simulink model "MyMOAB"  (R2021a)
settings: Solver=ode23t  StartTime=0.0  StopTime=Inf  RelTol=1e-3  AbsTol=1e-3
values from neighbouring files (symbols this model uses):
  ball_mass = DEFAULT_BALL_MASS    (= 0.0027)    [MOAB_PARAMS.m]
  ball_moi = calcMOI(ball_radius,ball_shell,ball_mass)    [MOAB_PARAMS.m]
  ball_radius = DEFAULT_BALL_RADIUS    (= 0.02)    [MOAB_PARAMS.m]
  ball_shell = DEFAULT_BALL_SHELL    (= 0.0002)    [MOAB_PARAMS.m]
  DEFAULT_BALL_NOISE = 0.0005    [MOAB_PARAMS.m]
  DEFAULT_GRAVITY = 9.81    [MOAB_PARAMS.m]
  DEFAULT_PLATE_NOISE = 0.0    (= 0)    [MOAB_PARAMS.m]
  DEFAULT_SIMULATION_RATE = 0.2    [MOAB_PARAMS.m]
  DEFAULT_VEL_NOISE = 0.0001    [MOAB_PARAMS.m]
  MAX_ITER = Inf    (= inf)    [MOAB_PARAMS.m]
  noise_mean = 0    [MOAB_PARAMS.m]
  noise_variance = 0.333    [MOAB_PARAMS.m]
  obstacle_radius = DEFAULT_OBSTACLE_RADIUS    (= 0)    [MOAB_PARAMS.m]
  plate_pos_z0 = DEFAULT_PLATE_HEIGHT    (= 0.02)    [MOAB_PARAMS.m]
  plate_radius = DEFAULT_PLATE_RADIUS    (= 0.1125)    [MOAB_PARAMS.m]
  s = 0.1732    [MOAB_PARAMS.m]
  target_pos_x = 0    [MOAB_PARAMS.m]
  target_pos_y = 0    [MOAB_PARAMS.m]
  tilt_acc = DEFAULT_PLATE_ANGULAR_ACCEL    [MOAB_PARAMS.m]
  tilt_limit = DEFAULT_PLATE_ANGLE_LIMIT    [MOAB_PARAMS.m]
  tilt_max_vel = DEFAULT_PLATE_MAX_ANGULAR_VELOCITY    [MOAB_PARAMS.m]
  tilt_x0 = deg2rad(0)    [MOAB_PARAMS.m]
  tilt_y0 = deg2rad(0)    [MOAB_PARAMS.m]
  TIME_DELTA = DEFAULT_SIMULATION_RATE    (= 0.2)    [MOAB_PARAMS.m]
  z_offset = 0.0328538    [MOAB_PARAMS.m]
undefined symbols (not defined in the file or in its folder): smiData, X, Y, Z
libraries: sm_lib x119, nesl_utility x21, simulink x1
(part 1 of 4)
settings Model: Creator=abiswas  LastModifiedBy=dbnun
settings SolverCC: AlgebraicLoopSolver=TrustRegion
settings DebuggingCC: InheritedTsInSrcMsg=none  SFMachineParentedDataDiag=warning
settings SimscapeCC: SimscapeLogType=all
settings DiagnosticsConfigSet: SimMechanicsUnsatisfiedHighPriorityTargets=none
settings ExplorerConfigSet: InternalSimMechanicsExplorerSettings="<ExplorerConfiguration><canonicalview>default</canonicalview><AnimationSetting><BasePlaybackSpeed>1.0</BasePlaybackSpeed><PlaybackSpeedFactor>1.0</PlaybackSpeedFactor></AnimationSetting><TilePanel><TileInfo><Tiles Columns=\"1\" Count=\"2\" Rows=\"2\"><Column Weight=\"1\"/><Row Weight=\"0.5678\"/><Row Weight=\"0.4322\"/><Tile Height=\"1\" Width=\"1\" X=\"0\" Y=\"0\"/><Tile Height=\"1\" Width=\"1\" X=\"0\" Y=\"1\"/></Tiles></TileInfo><SceneInfo><SceneViewer><BGColor><R>1</R><G>1</G><B>1</B></BGColor><Camera><DoPerspective>off</DoPerspective><Position><X>-0.0080012764069667501</X><Y>-0.00465270619968879105</Y><Z>1.03071236736211413</Z></Position><Center><X>-0.0080012764069667501</X><Y>-0.00465270619968879105</Y><Z>0.0307123673621141347</Z></Center><Up><X>-0.84666783086952091</X><Y>-0.532121775696785759</Y><Z>0</Z></Up><ViewLimDist>1</ViewLimDist><YLim>0.139428062443435197</YLim><XLim>0.213694846724530263</XLim></Camera></SceneViewer><SceneViewer><BGColor><R>1</R><G>1</G><B>1</B></BGColor><Camera><DoPerspective>off</DoPerspective><Position><X>0.994386182454623402</X><Y>0.0608673913546442444</Y><Z>0.0679676248852747467</Z></Position><Center><X>-0.00298892093291726986</X><Y>0.00143103908732779002</Y><Z>0.0266127802857842946</Z></Center><Up><X>-0.040438631297503691</X><Y>-0.0165365771902967751</Y><Z>0.999045173509994111</Z></Up><ViewLimDist>1</ViewLimDist><YLim>0.077297016049004505</YLim><XLim>0.156048545840866637</XLim></Camera></SceneViewer></SceneInfo></TilePanel><MechEditorPanel><Cameras/><GfxPanelCameraMap/><VideoCreator><PlaybackSpeedRatio>1.0</PlaybackSpeedRatio><FrameRate>30</FrameRate><VideoFormat>Motion JPEG AVI</VideoFormat><FrameSize>auto</FrameSize></VideoCreator></MechEditorPanel></ExplorerConfiguration>"

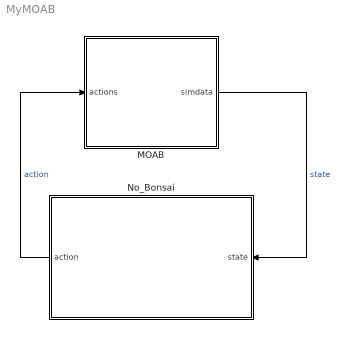
== system MyMOAB ==
  MOAB : Subsystem
      mask Display: image('MOAB_Full_IMAGE.png')
  No_Bonsai : Subsystem  VariantControl=Sinusoid
  wires:
  MOAB/1(simdata) -> No_Bonsai/1(state)  "state"
  No_Bonsai/1(action) -> MOAB/1(actions)  "action"

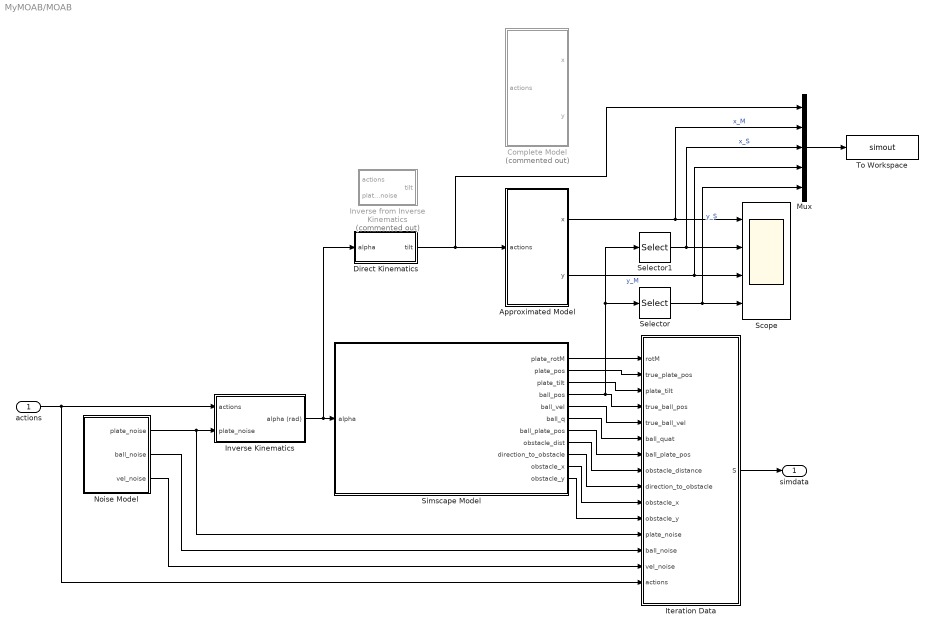
== system MyMOAB/MOAB ==
  actions : Inport
  Approximated Model : Subsystem
  Complete Model : Subsystem  Commented=on
  Direct Kinematics : Subsystem
  Inverse Kinematics : Subsystem
  Inverse from Inverse Kinematics : Subsystem  Commented=on
  Iteration Data : Subsystem  VariantControl=Choice
  Mux : Mux  Inputs=5
  Noise Model : Subsystem  Variant=on  VariantControlMode=label  LabelModeActiveChoice=Zero  mask{VChoice=Zero noise}
      mask prompts: VChoice "Noise model"
      mask init:
      | simulationStatus =  get_param(bdroot,'SimulationStatus');
      | 
      | % The active variant can only be modified at edit-time or very early during
      | % the simulink compile stage. 
      | 
      |     choice = get_param(gcb,'VChoice');
      |     vssBlk = gcb;
      |     oldVariant = get_param(gcb,'OverrideUsingVariant');
      | 
      |     if strcmp(choice,'Zero noise')
      | 
      |         set_param(vssBlk, 'OverrideUsingVariant', 'Zero');
      |     else
      | 
      |         set_param(vssBlk, 'OverrideUsingVariant', 'Gaussian');
      |     end
      mask TypeOptions VChoice: Zero noise | Gaussian noise
      mask DialogControl DescTextVar Prompt: Select a noise model for ball and plate states.
  Scope : Scope  NumInputPorts=4
  Selector : Selector  InputPortWidth=3  IndexOptions=Index vector (dialog)  Indices=[2]  OutputSizes=1
  Selector1 : Selector  InputPortWidth=3  IndexOptions=Index vector (dialog)  Indices=[1]  OutputSizes=1
  Simscape Model : Subsystem
      mask Display: image('MOAB_Full_IMAGE_small.png')
  To Workspace : ToWorkspace  VariableName=simout  SaveFormat=Timeseries  SampleTime=-1
  simdata : Outport
  wires:
  Inverse Kinematics/1(alpha (rad)) -> Direct Kinematics/1(alpha), Simscape Model/1(alpha)
  Noise Model/1(plate_noise) -> Inverse Kinematics/2(plate_noise), Iteration Data/12(plate_noise)
  Iteration Data/1(S) -> simdata/1
  Noise Model/2(ball_noise) -> Iteration Data/13(ball_noise)
  Noise Model/3(vel_noise) -> Iteration Data/14(vel_noise)
  Simscape Model/7(ball_plate_pos) -> Iteration Data/7(ball_plate_pos)
  Simscape Model/6(ball_q) -> Iteration Data/6(ball_quat)
  Simscape Model/5(ball_vel) -> Iteration Data/5(true_ball_vel)
  Simscape Model/4(ball_pos) -> Selector1/1, Selector/1, Iteration Data/4(true_ball_pos)
  Simscape Model/2(plate_pos) -> Iteration Data/2(true_plate_pos)
  Simscape Model/1(plate_rotM) -> Iteration Data/1(rotM)
  Simscape Model/8(obstacle_dist) -> Iteration Data/8(obstacle_distance)
  Simscape Model/3(plate_tilt) -> Iteration Data/3(plate_tilt)
  Simscape Model/9(direction_to_obstacle) -> Iteration Data/9(direction_to_obstacle)
  Simscape Model/10(obstacle_x) -> Iteration Data/10(obstacle_x)
  Simscape Model/11(obstacle_y) -> Iteration Data/11(obstacle_y)
  Selector/1 -> Mux/5, Scope/4  "y_S"
  Selector1/1 -> Mux/3, Scope/2  "x_S"
  actions/1 -> Iteration Data/15(actions), Inverse Kinematics/1(actions)
  Approximated Model/2(y) -> Mux/4, Scope/3  "y_M"
  Approximated Model/1(x) -> Mux/2, Scope/1  "x_M"
  Direct Kinematics/1(tilt) -> Mux/1, Approximated Model/1(actions)
  Mux/1 -> To Workspace/1

== system MyMOAB/No_Bonsai ==
  state : Inport
  Constant1 : Constant  Value=false
  "Sinusoidal " : Subsystem
  Stop Simulation1 : Stop
  action : Outport
  wires:
  Constant1/1 -> "Sinusoidal "/2(halted)
  "Sinusoidal "/2(reset) -> Stop Simulation1/1
  state/1 -> "Sinusoidal "/1(state)
  "Sinusoidal "/1(actions) -> action/1

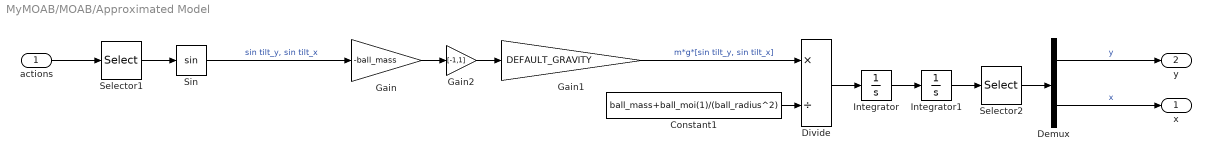
== system MyMOAB/MOAB/Approximated Model ==
  actions : Inport
  Constant1 : Constant  Value=ball_mass+ball_moi(1)/(ball_radius^2)
  Demux : Demux  Outputs=2
  Divide : Product  Inputs=*/
  Gain : Gain  Gain=-ball_mass
  Gain1 : Gain  Gain=DEFAULT_GRAVITY
  Gain2 : Gain  Gain=[-1,1]
  Integrator : Integrator
  Integrator1 : Integrator
  Selector1 : Selector  InputPortWidth=2  IndexOptions=Index vector (dialog)  Indices=[2 1]  OutputSizes=1
  Selector2 : Selector  InputPortWidth=2  IndexOptions=Index vector (dialog)  Indices=[2 1]  OutputSizes=1
  Sin : Trigonometry
  x : Outport
  y : Outport  Port=2
  wires:
  Divide/1 -> Integrator/1
  Integrator/1 -> Integrator1/1
  Demux/2 -> x/1  "x"
  Gain1/1 -> Divide/1  "m*g*[sin tilt_y, sin tilt_x]"
  Selector1/1 -> Sin/1
  Demux/1 -> y/1  "y"
  Integrator1/1 -> Selector2/1
  Selector2/1 -> Demux/1
  actions/1 -> Selector1/1
  Constant1/1 -> Divide/2
  Sin/1 -> Gain/1  "sin tilt_y, sin tilt_x"
  Gain/1 -> Gain2/1
  Gain2/1 -> Gain1/1

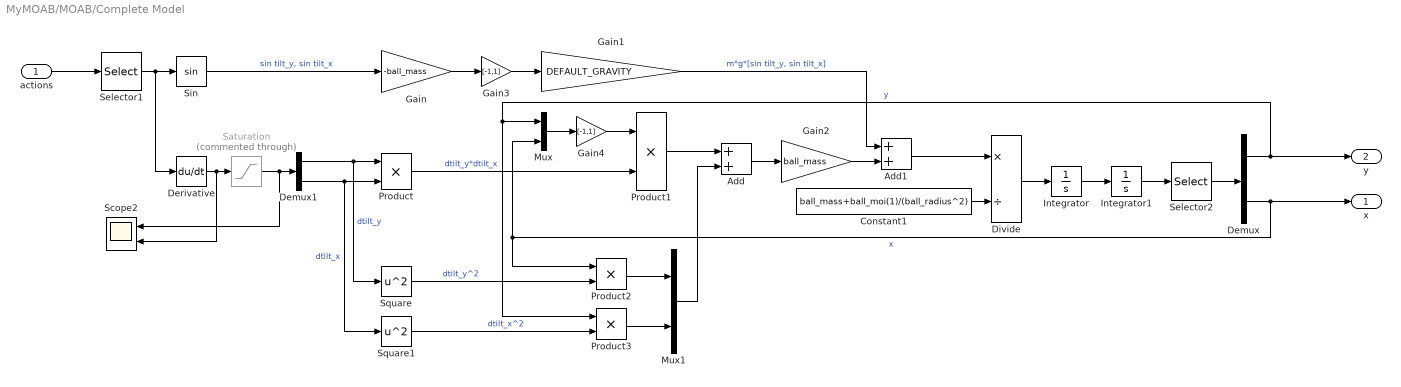
== system MyMOAB/MOAB/Complete Model ==
  actions : Inport
  Add : Sum
  Add1 : Sum
  Constant1 : Constant  Value=ball_mass+ball_moi(1)/(ball_radius^2)
  Demux : Demux  Outputs=2
  Demux1 : Demux  Outputs=2
  Derivative : Derivative
  Divide : Product  Inputs=*/
  Gain : Gain  Gain=-ball_mass
  Gain1 : Gain  Gain=DEFAULT_GRAVITY
  Gain2 : Gain  Gain=ball_mass
  Gain3 : Gain  Gain=[-1,1]
  Gain4 : Gain  Gain=[-1,1]
  Integrator : Integrator
  Integrator1 : Integrator
  Mux : Mux  Inputs=2
  Mux1 : Mux  Inputs=2
  Product{,1..3} (4 alike) : Product
  Saturation : Saturate  Commented=through  UpperLimit=50  LowerLimit=-50
  Scope2 : Scope  NumInputPorts=2
  Selector1 : Selector  InputPortWidth=2  IndexOptions=Index vector (dialog)  Indices=[2 1]  OutputSizes=1
  Selector2 : Selector  InputPortWidth=2  IndexOptions=Index vector (dialog)  Indices=[2 1]  OutputSizes=1
  Sin : Trigonometry
  Square : Math  Operator=square  SaturateOnIntegerOverflow=on
  Square1 : Math  Operator=square  SaturateOnIntegerOverflow=on
  x : Outport
  y : Outport  Port=2
  wires:
  Demux1/2 -> Square1/1, Product/2  "dtilt_x"
  Add/1 -> Gain2/1
  Square/1 -> Product2/2  "dtilt_y^2"
  Square1/1 -> Product3/2  "dtilt_x^2"
  Mux1/1 -> Add/2
  Derivative/1 -> Scope2/2, Saturation/1
  Product2/1 -> Mux1/1
  Gain2/1 -> Add1/2
  Divide/1 -> Integrator/1
  Integrator/1 -> Integrator1/1
  Product1/1 -> Add/1
  Demux1/1 -> Square/1, Product/1  "dtilt_y"
  Add1/1 -> Divide/1
  Demux/2 -> x/1, Mux/2, Product2/1  "x"
  Gain1/1 -> Add1/1  "m*g*[sin tilt_y, sin tilt_x]"
  Gain/1 -> Gain3/1
  Mux/1 -> Gain4/1
  Product/1 -> Product1/2  "dtilt_y*dtilt_x"
  Saturation/1 -> Scope2/1, Demux1/1
  Selector1/1 -> Sin/1, Derivative/1
  Demux/1 -> y/1, Product3/1, Mux/1  "y"
  Integrator1/1 -> Selector2/1
  Selector2/1 -> Demux/1
  actions/1 -> Selector1/1
  Constant1/1 -> Divide/2
  Product3/1 -> Mux1/2
  Sin/1 -> Gain/1  "sin tilt_y, sin tilt_x"
  Gain3/1 -> Gain1/1
  Gain4/1 -> Product1/1

== system MyMOAB/MOAB/Direct Kinematics ==
  alpha : Inport
  Constant : Constant  Value=plate_pos_z0+z_offset
  MATLAB Function : MATLAB Function  TreatAsAtomicUnit=on
  tilt : Outport
  wires:
  Constant/1 -> MATLAB Function/2(h)
  alpha/1 -> MATLAB Function/1(alpha)
  MATLAB Function/1(tilt) -> tilt/1

== system MyMOAB/MOAB/Inverse Kinematics ==
  note: Generate approximate servo angles from plate height and tilt angles.
  actions : Inport
  plate_noise : Inport  Port=2
  Constant : Constant  Value=plate_pos_z0+z_offset
  Convert To Tilt Angles : Gain  Gain=tilt_limit
  Demux : Demux  Outputs=2
  MATLAB Function : MATLAB Function  TreatAsAtomicUnit=on
  Reshape : Reshape
  alpha (rad) : Outport
  wires:
  Demux/2 -> MATLAB Function/3(tilt_y)  "(rad)"
  Demux/1 -> MATLAB Function/2(tilt_x)  "(rad)"
  MATLAB Function/1(alpha) -> Reshape/1
  Constant/1 -> MATLAB Function/1(plate_height)
  Reshape/1 -> alpha (rad)/1
  plate_noise/1 -> MATLAB Function/4(plate_noise)
  actions/1 -> Convert To Tilt Angles/1
  Convert To Tilt Angles/1 -> Demux/1

== system MyMOAB/MOAB/Inverse from Inverse Kinematics ==
  actions : Inport
  plate_noise : Inport  Port=2
  Convert To Tilt Angles : Gain  Gain=tilt_limit
  Sum : Sum  Inputs=|++
  tilt : Outport
  wires:
  Convert To Tilt Angles/1 -> Sum/1
  actions/1 -> Convert To Tilt Angles/1
  plate_noise/1 -> Sum/2
  Sum/1 -> tilt/1

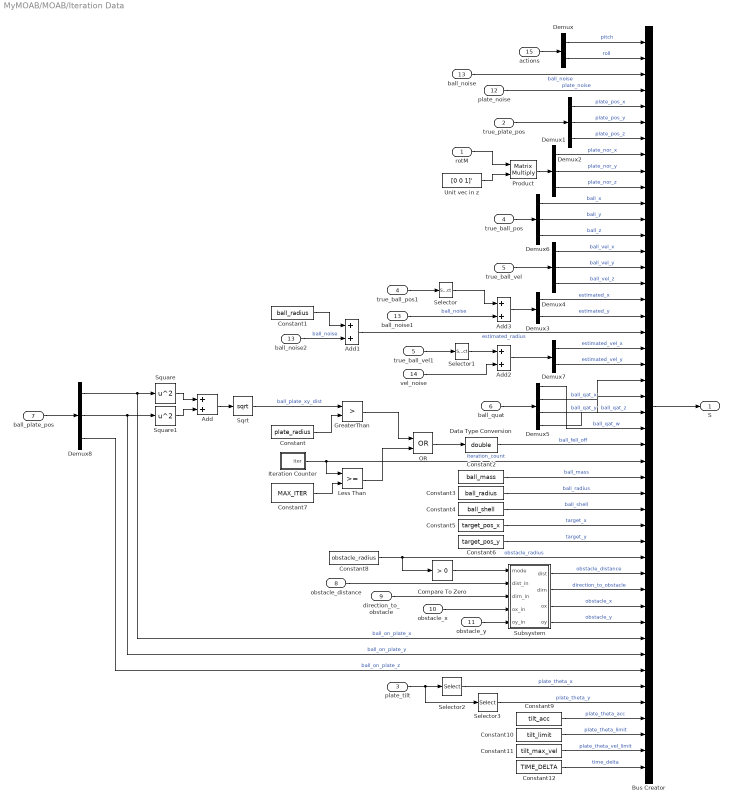
== system MyMOAB/MOAB/Iteration Data ==
  rotM : Inport
  true_plate_pos : Inport  Port=2
  plate_tilt : Inport  Port=3
  true_ball_pos : Inport  Port=4
  true_ball_vel : Inport  Port=5
  ball_quat : Inport  Port=6
  ball_plate_pos : Inport  Port=7
  obstacle_distance : Inport  Port=8
  direction_to_obstacle : Inport  Port=9
  obstacle_x : Inport  Port=10
  obstacle_y : Inport  Port=11
  plate_noise : Inport  Port=12
  ball_noise : Inport  Port=13
  vel_noise : Inport  Port=14
  actions : Inport  Port=15
  Add{,1..3} (4 alike) : Sum
  Bus Creator : BusCreator  Inputs=46
  Compare To Zero : simulink/Logic and Bit Operations/Compare To Zero  relop=>  OutDataTypeStr=boolean
  Constant : Constant  Value=plate_radius
  Constant1 : Constant  Value=ball_radius
  Constant10 : Constant  Value=tilt_limit
  Constant11 : Constant  Value=tilt_max_vel
  Constant12 : Constant  Value=TIME_DELTA
  Constant2 : Constant  Value=ball_mass
  Constant3 : Constant  Value=ball_radius
  Constant4 : Constant  Value=ball_shell
  Constant5 : Constant  Value=target_pos_x
  Constant6 : Constant  Value=target_pos_y
  Constant7 : Constant  Value=MAX_ITER
  Constant8 : Constant  Value=obstacle_radius
  Constant9 : Constant  Value=tilt_acc
  Data Type Conversion : DataTypeConversion  OutDataTypeStr=double
  Demux : Demux  Outputs=2
  Demux{1..2,4,6,8} (5 alike) : Demux  Outputs=3
  Demux3 : Demux  Outputs=2
  Demux5 : Demux
  Demux7 : Demux  Outputs=2
  GreaterThan : RelationalOperator  Operator=>  OutDataTypeStr=boolean  RndMeth=Simplest
  Iteration Counter : Subsystem
  Less Than : RelationalOperator  OutDataTypeStr=boolean  RndMeth=Simplest
  OR : Logic  Operator=OR  AllPortsSameDT=off  OutDataTypeStr=boolean
  Product : Product  Multiplication=Matrix(*)
  Selector : Selector  InputPortWidth=3  IndexOptions=Index vector (dialog)  Indices=1:2  OutputSizes=1
  Selector1 : Selector  InputPortWidth=3  IndexOptions=Index vector (dialog)  Indices=1:2  OutputSizes=1
  Selector2 : Selector  InputPortWidth=3  IndexOptions=Index vector (dialog)  Indices=1  OutputSizes=1
  Selector3 : Selector  InputPortWidth=3  IndexOptions=Index vector (dialog)  Indices=2  OutputSizes=1
  Sqrt : Sqrt  SaturateOnIntegerOverflow=on
  Square : Math  Operator=square  SaturateOnIntegerOverflow=on
  Square1 : Math  Operator=square  SaturateOnIntegerOverflow=on
  Subsystem : Subsystem
  Unit vec in z : Constant  Value=[0 0 1]'
  ball_noise1 : InportShadow  Port=13
  ball_noise2 : InportShadow  Port=13
  true_ball_pos1 : InportShadow  Port=4
  true_ball_vel1 : InportShadow  Port=5
  S : Outport
  wires:
  Demux3/2 -> Bus Creator/18  "estimated_y"
  true_ball_pos/1 -> Demux6/1
  Demux2/1 -> Bus Creator/5  "plate_pos_x"
  Demux5/3 -> Bus Creator/23  "ball_qat_y"
  Demux5/1 -> Bus Creator/25  "ball_qat_w"
  Product/1 -> Demux1/1
  Demux4/1 -> Bus Creator/14  "ball_vel_x"
  Demux5/2 -> Bus Creator/22  "ball_qat_x"
  Demux1/2 -> Bus Creator/9  "plate_nor_y"
  Demux2/3 -> Bus Creator/7  "plate_pos_z"
  Unit vec in z/1 -> Product/2
  rotM/1 -> Product/1
  Demux2/2 -> Bus Creator/6  "plate_pos_y"
  Demux/1 -> Bus Creator/1  "pitch"
  Constant10/1 -> Bus Creator/44  "plate_theta_limit"
  Add3/1 -> Demux3/1
  Iteration Counter/1(iter) -> Less Than/1, Bus Creator/27  "iteration_count"
  Subsystem/4(oy) -> Bus Creator/37  "obstacle_y"
  Demux8/3 -> Bus Creator/40  "ball_on_plate_z"
  true_ball_vel1/1 -> Selector1/1
  Demux5/4 -> Bus Creator/24  "ball_qat_z"
  Square1/1 -> Add/2
  ball_noise2/1 -> Add1/2  "ball_noise"
  Constant6/1 -> Bus Creator/32  "target_y"
  true_ball_pos1/1 -> Selector/1
  Constant5/1 -> Bus Creator/31  "target_x"
  Constant2/1 -> Bus Creator/28  "ball_mass"
  plate_noise/1 -> Bus Creator/4  "plate_noise"
  Constant/1 -> GreaterThan/2
  GreaterThan/1 -> OR/1
  Data Type Conversion/1 -> Bus Creator/26  "ball_fell_off"
  Add2/1 -> Demux7/1
  true_ball_vel/1 -> Demux4/1
  true_plate_pos/1 -> Demux2/1
  OR/1 -> Data Type Conversion/1
  Demux3/1 -> Bus Creator/17  "estimated_x"
  Demux4/2 -> Bus Creator/15  "ball_vel_y"
  Bus Creator/1 -> S/1
  Demux4/3 -> Bus Creator/16  "ball_vel_z"
  Subsystem/3(ox) -> Bus Creator/36  "obstacle_x"
  Demux6/2 -> Bus Creator/12  "ball_y"
  Less Than/1 -> OR/2
  Add/1 -> Sqrt/1
  Subsystem/2(dirn) -> Bus Creator/35  "direction_to_obstacle"
  Constant11/1 -> Bus Creator/45  "plate_theta_vel_limit"
  Demux1/3 -> Bus Creator/10  "plate_nor_z"
  Subsystem/1(dist) -> Bus Creator/34  "obstacle_distance"
  Constant3/1 -> Bus Creator/29  "ball_radius"
  Constant12/1 -> Bus Creator/46  "time_delta"
  vel_noise/1 -> Add2/2
  Selector2/1 -> Bus Creator/41  "plate_theta_x"
  Sqrt/1 -> GreaterThan/1  "ball_plate_xy_dist"
  Demux7/1 -> Bus Creator/20  "estimated_vel_x"
  Constant8/1 -> Bus Creator/33, Compare To Zero/1  "obstacle_radius"
  Square/1 -> Add/1
  actions/1 -> Demux/1
  Selector3/1 -> Bus Creator/42  "plate_theta_y"
  Demux/2 -> Bus Creator/2  "roll"
  ball_noise/1 -> Bus Creator/3  "ball_noise"
  Demux6/1 -> Bus Creator/11  "ball_x"
  plate_tilt/1 -> Selector3/1, Selector2/1
  Constant7/1 -> Less Than/2
  Selector/1 -> Add3/1
  Constant9/1 -> Bus Creator/43  "plate_theta_acc"
  Demux6/3 -> Bus Creator/13  "ball_z"
  Add1/1 -> Bus Creator/19  "estimated_radius"
  Demux1/1 -> Bus Creator/8  "plate_nor_x"
  Demux8/1 -> Square/1, Bus Creator/38  "ball_on_plate_x"
  ball_plate_pos/1 -> Demux8/1
  Demux7/2 -> Bus Creator/21  "estimated_vel_y"
  Selector1/1 -> Add2/1
  Constant4/1 -> Bus Creator/30  "ball_shell"
  ball_noise1/1 -> Add3/2  "ball_noise"
  Constant1/1 -> Add1/1
  ball_quat/1 -> Demux5/1
  Demux8/2 -> Square1/1, Bus Creator/39  "ball_on_plate_y"
  Compare To Zero/1 -> Subsystem/1(mode)
  obstacle_distance/1 -> Subsystem/2(dist_in)
  direction_to_obstacle/1 -> Subsystem/3(dirn_in)
  obstacle_x/1 -> Subsystem/4(ox_in)
  obstacle_y/1 -> Subsystem/5(oy_in)

== system MyMOAB/MOAB/Noise Model ==
  note: 1) Add Subsystem or Model blocks as valid variant choices.
      | 2) You cannot connect blocks at this level. At simulation, connectivity is automatically
      | determined, based on the active variant and port name matching.
  Gaussian Noise : Subsystem  VariantControl=Gaussian
  Zero Noise : Subsystem  VariantControl=Zero
  plate_noise : Outport
  ball_noise : Outport  Port=2
  vel_noise : Outport  Port=3

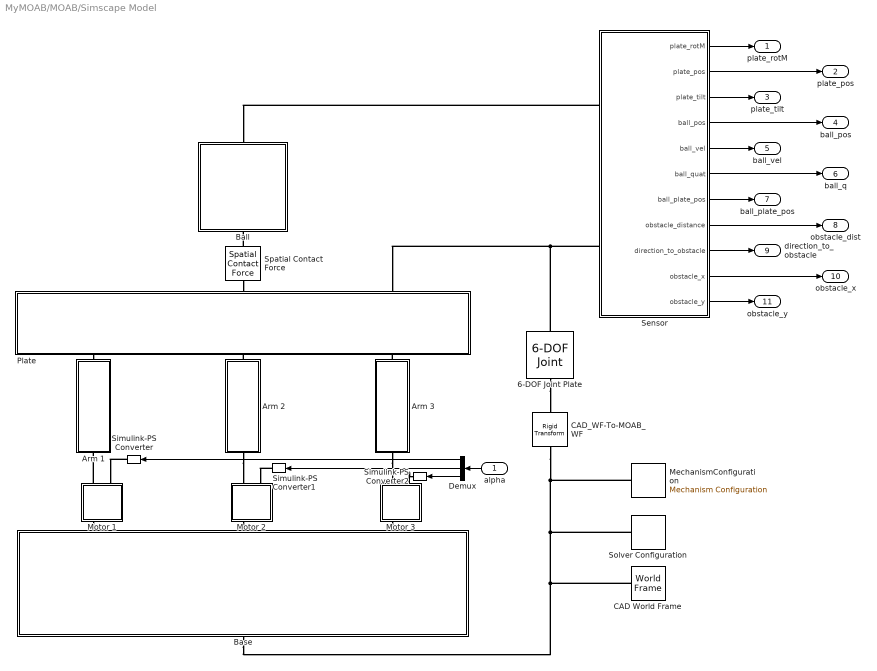
== system MyMOAB/MOAB/Simscape Model ==
  alpha : Inport
  6-DOF Joint Plate : sm_lib/Joints/6-DOF Joint  JointMode=Normal  SenseConstraintForce=off  SenseConstraintForceX=off  SenseConstraintForceY=off  SenseConstraintForceZ=off  SenseConstraintTorque=off  SenseConstraintTorqueX=off  SenseConstraintTorqueY=off  SenseConstraintTorqueZ=off  SenseTotalForce=off  SenseTotalForceX=off  SenseTotalForceY=off  SenseTotalForceZ=off  SenseTotalTorque=off  SenseTotalTorqueX=off  SenseTotalTorqueY=off  SenseTotalTorqueZ=off  CompositeWrenchDir=FollowerOnBase  CompositeWrenchFrame=BaseFrame  PxEquilibriumPosition=0  PxEquilibriumPositionUnits=m  PxSpringStiffness=0  PxSpringStiffnessUnits=N/m  PxDampingCoefficient=0  PxDampingCoefficientUnits=N/(m/s)  PxTorqueActuationMode=NoTorque  PxMotionActuationMode=ComputedMotion  PxSensePosition=off  PxSenseVelocity=off  PxSenseAcceleration=off  PxSenseTorqueForce=off  PxSenseLowerLimitTorqueForce=off  PxSenseUpperLimitTorqueForce=off  PxLowerLimitSpecify=off  PxLowerLimitBound=-1  PxLowerLimitBoundUnits=m  PxLowerLimitStiffness=1e6  PxLowerLimitStiffnessUnits=N/m  PxLowerLimitDamping=1e3  PxLowerLimitDampingUnits=N/(m/s)  PxLowerLimitTransitionRegionWidth=1e-4  PxLowerLimitTransitionRegionWidthUnits=m  PxUpperLimitSpecify=off  PxUpperLimitBound=1  PxUpperLimitBoundUnits=m  PxUpperLimitStiffness=1e6  PxUpperLimitStiffnessUnits=N/m  PxUpperLimitDamping=1e3  PxUpperLimitDampingUnits=N/(m/s)  PxUpperLimitTransitionRegionWidth=1e-4  PxUpperLimitTransitionRegionWidthUnits=m  PxPositionTargetSpecify=on  PxPositionTargetPriority=Low  PxPositionTargetValue=0  PxPositionTargetValueUnits=m  PxVelocityTargetSpecify=off  PxVelocityTargetPriority=High  PxVelocityTargetValue=0  PxVelocityTargetValueUnits=m/s  PyEquilibriumPosition=0  PyEquilibriumPositionUnits=m  PySpringStiffness=0  PySpringStiffnessUnits=N/m  PyDampingCoefficient=0  PyDampingCoefficientUnits=N/(m/s)  PyTorqueActuationMode=NoTorque  PyMotionActuationMode=ComputedMotion  PySensePosition=off  PySenseVelocity=off  PySenseAcceleration=off  PySenseTorqueForce=off  PySenseLowerLimitTorqueForce=off  PySenseUpperLimitTorqueForce=off  PyLowerLimitSpecify=off  PyLowerLimitBound=0  PyLowerLimitBoundUnits=m  PyLowerLimitStiffness=1e6  PyLowerLimitStiffnessUnits=N/m  PyLowerLimitDamping=1e3  PyLowerLimitDampingUnits=N/(m/s)  PyLowerLimitTransitionRegionWidth=1e-4  PyLowerLimitTransitionRegionWidthUnits=m  PyUpperLimitSpecify=off  PyUpperLimitBound=0  PyUpperLimitBoundUnits=m  PyUpperLimitStiffness=1e6  PyUpperLimitStiffnessUnits=N/m  PyUpperLimitDamping=1e3  PyUpperLimitDampingUnits=N/(m/s)  PyUpperLimitTransitionRegionWidth=1e-4  PyUpperLimitTransitionRegionWidthUnits=m  PyPositionTargetSpecify=on  PyPositionTargetPriority=Low  PyPositionTargetValue=0  PyPositionTargetValueUnits=m  PyVelocityTargetSpecify=off  PyVelocityTargetPriority=High  PyVelocityTargetValue=0  PyVelocityTargetValueUnits=m/s  PzEquilibriumPosition=0  PzEquilibriumPositionUnits=m  PzSpringStiffness=0  PzSpringStiffnessUnits=N/m  PzDampingCoefficient=0  PzDampingCoefficientUnits=N/(m/s)  PzTorqueActuationMode=NoTorque  PzMotionActuationMode=ComputedMotion  PzSensePosition=off  PzSenseVelocity=off  PzSenseAcceleration=off  PzSenseTorqueForce=off  PzSenseLowerLimitTorqueForce=off  PzSenseUpperLimitTorqueForce=off  PzLowerLimitSpecify=on  PzLowerLimitBound=plate_zmin  PzLowerLimitBoundUnits=m  PzLowerLimitStiffness=1e6  PzLowerLimitStiffnessUnits=N/m  PzLowerLimitDamping=1e3  PzLowerLimitDampingUnits=N/(m/s)  PzLowerLimitTransitionRegionWidth=1e-4  PzLowerLimitTransitionRegionWidthUnits=m  PzUpperLimitSpecify=on  PzUpperLimitBound=plate_zmax  PzUpperLimitBoundUnits=m  PzUpperLimitStiffness=1e6  PzUpperLimitStiffnessUnits=N/m  PzUpperLimitDamping=1e3  PzUpperLimitDampingUnits=N/(m/s)  PzUpperLimitTransitionRegionWidth=1e-4  PzUpperLimitTransitionRegionWidthUnits=m  PzPositionTargetSpecify=on  PzPositionTargetPriority=High  PzPositionTargetValue=plate_pos_z0  PzPositionTargetValueUnits=m  PzVelocityTargetSpecify=off  PzVelocityTargetPriority=High  PzVelocityTargetValue=0  PzVelocityTargetValueUnits=m/s  SphDefPosRotationMethod=None  SphDefPosRotationAngleUnits=deg  SphDefPosRotationStandardAxis=+Z  SphDefPosRotationAngle=0.0  SphDefPosRotationArbitraryAxis=[0 0 1]  SphDefPosFollAlignAxisA=+X  SphDefPosBaseAlignAxisA=+Y  SphDefPosFollAlignAxisB=+Y  SphDefPosBaseAlignAxisB=+Z  SphDefPosRotationSequenceAxes=FollowerAxes  SphDefPosRotationSequence=XYX  SphDefPosRotationSequenceAngles=[0 0 0]  SphDefPosRotationSequenceAnglesUnits=deg  SphDefPosRotationMatrix=[1 0 0; 0 1 0; 0 0 1]  SphEqPosRotationMethod=None  SphEqPosRotationAngleUnits=deg  SphEqPosRotationStandardAxis=+Z  SphEqPosRotationAngle=0.0  SphEqPosRotationArbitraryAxis=[0 0 1]  SphEqPosFollAlignAxisA=+X  SphEqPosBaseAlignAxisA=+Y  SphEqPosFollAlignAxisB=+Y  SphEqPosBaseAlignAxisB=+Z  SphEqPosRotationSequenceAxes=FollowerAxes  SphEqPosRotationSequence=XYX  SphEqPosRotationSequenceAngles=[0 0 0]  SphEqPosRotationSequenceAnglesUnits=deg  SphEqPosRotationMatrix=[1 0 0; 0 1 0; 0 0 1]  SphSpringStiffness=0  SphSpringStiffnessUnits=N*m/deg  SphDampingCoefficient=0  SphDampingCoefficientUnits=N*m/(deg/s)  SphActuateTorqueX=off  SphActuateTorqueY=off  SphActuateTorqueZ=off  SphActuateTorque=off  SphTorqueActuationMode=NoTorque  SphMotionActuationMode=ComputedMotion  SphActuationFrame=BaseFrame  SphSensePosition=off  SphSenseVelocityX=off  SphSenseVelocityY=off  SphSenseVelocityZ=off  SphSenseVelocity=off  SphSenseAccelerationX=off  SphSenseAccelerationY=off  SphSenseAccelerationZ=off  SphSenseAcceleration=off  SphSenseTorqueX=off  SphSenseTorqueY=off  SphSenseTorqueZ=off  SphSenseTorqueForce=off  SphSenseLowerLimitTorqueMag=off  SphSenseUpperLimitTorqueMag=off  SphSensingFrame=BaseFrame  SphLowerLimitSpecify=off  SphLowerLimitBound=-tilt_limit  SphLowerLimitBoundUnits=rad  SphLowerLimitStiffness=1e4  SphLowerLimitStiffnessUnits=N*m/deg  SphLowerLimitDamping=10  SphLowerLimitDampingUnits=N*m/(deg/s)  SphLowerLimitTransitionRegionWidth=0.1  SphLowerLimitTransitionRegionWidthUnits=deg  SphUpperLimitSpecify=off  SphUpperLimitBound=tilt_limit  SphUpperLimitBoundUnits=rad  SphUpperLimitStiffness=1e4  SphUpperLimitStiffnessUnits=N*m/deg  SphUpperLimitDamping=10  SphUpperLimitDampingUnits=N*m/(deg/s)  SphUpperLimitTransitionRegionWidth=0.1  SphUpperLimitTransitionRegionWidthUnits=deg  SphPositionTargetRotationMethod=RotationSequence  SphPositionTargetRotationAngleUnits=deg  SphPositionTargetRotationStandardAxis=+X  SphPositionTargetRotationAngle=0.0  SphPositionTargetRotationArbitraryAxis=[0 0 1]  SphPositionTargetFollAlignAxisA=+X  SphPositionTargetBaseAlignAxisA=+Y  SphPositionTargetFollAlignAxisB=+Y  SphPositionTargetBaseAlignAxisB=+Z  SphPositionTargetRotationSequenceAxes=FollowerAxes  SphPositionTargetRotationSequence=XYZ  SphPositionTargetRotationSequenceAngles=[tilt_y0 tilt_x0 0]  SphPositionTargetRotationSequenceAnglesUnits=rad  SphPositionTargetRotationMatrix=eye(3)  SphPositionTargetSpecify=on  SphPositionTargetPriority=High  SphVelocityTargetValue=[0 0 0]  SphVelocityTargetValueUnits=deg/s  SphVelocityTargetSpecify=off  SphVelocityTargetPriority=High  SphVelocityTargetInFollowerFrame=on
  Arm 1 : Subsystem
      mask Display: image('MOAB_Arm_IMAGE.png')
  Arm 2 : Subsystem
      mask Display: image('MOAB_Arm_IMAGE.png')
  Arm 3 : Subsystem
      mask Display: image('MOAB_Arm_IMAGE.png')
  Ball : Subsystem
      mask Display: image('MOAB_Ball_IMAGE.png');
  Base : Subsystem
      mask Display: image('MOAB_Base_IMAGE.png');
  CAD World Frame : sm_lib/Frames and Transforms/World Frame
  CAD_WF-To-MOAB_WF : sm_lib/Frames and Transforms/Rigid Transform  TranslationMethod=StandardAxis  TranslationStandardOffset=z_offset  TranslationLengthUnit=m  TranslationStandardAxis=+Z  TranslationCartesianOffset=[0 0 0]  TranslationROffset=0  TranslationROffsetUnits=m  TranslationZOffset=0  TranslationZOffsetUnits=m  TranslationThetaOffset=0  TranslationThetaOffsetUnits=deg  RotationMethod=None  RotationAngleUnits=deg  RotationStandardAxis=+Z  RotationAngle=0.0  RotationArbitraryAxis=[0 0 1]  FollAlignAxisA=+X  BaseAlignAxisA=+Y  FollAlignAxisB=+Y  BaseAlignAxisB=+Z  RotationSequenceAxes=FollowerAxes  RotationSequence=XYX  RotationSequenceAngles=[0 0 0]  RotationSequenceAnglesUnits=deg  RotationMatrix=[1 0 0; 0 1 0; 0 0 1]
  Demux : Demux  Outputs=3
  MechanismConfiguration : sm_lib/Utilities/Mechanism Configuration  UniformGravity=Constant  GravityVector=[0 0 -DEFAULT_GRAVITY]  GravityVectorUnits=m/s^2  GravityUnits=m/s^2  LinearizationDelta=0.001  JointModeTransitionNonlinearIterations=2
  Motor 1 : Subsystem
  Motor 2 : Subsystem
  Motor 3 : Subsystem
  Plate : Subsystem
      mask Display: image('MOAB_Plate_IMAGE.png');
  Sensor : Subsystem
  Simulink-PS Converter : nesl_utility/Simulink-PS Converter  PhysicalDomain=network_engine_domain  SubClassName=ps_input  LeftPortType=input  RightPortType=output  PseudoPeriodic=off  Frequencies=[]  NoiseDistribution=none  NoiseParameters=[]  Unit=rad  AffineConversion=off  FilteringAndDerivatives=filter  SimscapeFilterOrder=2  InputFilterTimeConstant=0.01  UdotUserProvided=0
      settings: SourceProductBaseCode=PW,SS
  Simulink-PS Converter1 : nesl_utility/Simulink-PS Converter  PhysicalDomain=network_engine_domain  SubClassName=ps_input  LeftPortType=input  RightPortType=output  PseudoPeriodic=off  Frequencies=[]  NoiseDistribution=none  NoiseParameters=[]  Unit=rad  AffineConversion=off  FilteringAndDerivatives=filter  SimscapeFilterOrder=2  InputFilterTimeConstant=0.01  UdotUserProvided=0
      settings: SourceProductBaseCode=PW,SS
  Simulink-PS Converter2 : nesl_utility/Simulink-PS Converter  PhysicalDomain=network_engine_domain  SubClassName=ps_input  LeftPortType=input  RightPortType=output  PseudoPeriodic=off  Frequencies=[]  NoiseDistribution=none  NoiseParameters=[]  Unit=rad  AffineConversion=off  FilteringAndDerivatives=filter  SimscapeFilterOrder=2  InputFilterTimeConstant=0.01  UdotUserProvided=0
      settings: SourceProductBaseCode=PW,SS
  Solver Configuration : nesl_utility/Solver Configuration  PhysicalDomain=network_engine_domain  SubClassName=solver  LeftPortType=input  RightPortType=generic  Tones=[]  Harmonics=[]  SimulateNoise=off  Profile=off  UseLocalSampling=off  EnableSwitchedLinearOptims=on  FrequencyDomain=off  UseCCode=off  RelTol=0.001  AbsTol=1e-06  MinStep=1e-09  ToWorkspace=off  RevertToSquareIcSolve=off  NumHomotopyIterations=100  PhasorMode=off  PhasorModeNumHarmonics=1  DoDC=off  ResidualTolerance=1e-09  UseLocalSolver=off  LocalSolverChoice=NE_BACKWARD_EULER_ADVANCER  LocalSolverSampleTime=0.001  DoFixedCost=off  MaxNonlinIter=3  MaxModeIter=2  ComputeImpulses=off  ImpulseIterations=2  LinearAlgebra=Sparse  EquationFormulation=NE_TIME_EF  DelaysMemoryBudget=1024  AutomaticFiltering=on  FilteringTimeConstant=0.001  PartitionStorageMethod=AS_NEEDED  PartitionMemoryBudget=1024  PartitionMethod=ROBUST
      settings: SourceProductBaseCode=PW,SS
  Spatial Contact Force : sm_lib/Forces and Torques/Spatial Contact Force  CoefficientOfDynamicFriction=ball_dynamicfriction  CoefficientOfStaticFriction=ball_staticfriction  SenseContactBaseRotation=off  SenseContactBaseTranslation=off  NormalDamping=ball_damping  NormalDampingUnits=N/(m/s)  SenseContactFollowerRotation=off  SenseContactFollowerTranslation=off  SenseContactSignal=off  NormalStiffness=ball_stiffness  NormalStiffnessUnits=N/m  FrictionalCriticalVelocity=ball_criticalvelocity  FrictionalCriticalVelocityUnits=m/s  ZeroCrossDetectContactStartAndEnd=off  FrictionType=SmoothStickSlip  SenseFrictionalForceMagnitude=off  SenseNormalForceMagnitude=off  NormalForceType=SmoothSpringDamper  SenseNormalVelocity=off  SenseSeparationDistance=off  SenseTangentialVelocity=off  SenseTangentialVelocityMagnitude=off  NormalTransitionRegionWidth=ball_transitionwidth  NormalTransitionRegionWidthUnits=m
  plate_rotM : Outport
  plate_pos : Outport  Port=2
  plate_tilt : Outport  Port=3
  ball_pos : Outport  Port=4
  ball_vel : Outport  Port=5
  ball_q : Outport  Port=6
  ball_plate_pos : Outport  Port=7
  obstacle_dist : Outport  Port=8
  direction_to_obstacle : Outport  Port=9
  obstacle_x : Outport  Port=10
  obstacle_y : Outport  Port=11
  wires:
  Demux/3 -> Simulink-PS Converter2/1
  Demux/2 -> Simulink-PS Converter1/1
  Sensor/4(ball_pos) -> ball_pos/1
  Sensor/5(ball_vel) -> ball_vel/1
  Sensor/6(ball_quat) -> ball_q/1
  alpha/1 -> Demux/1
  Demux/1 -> Simulink-PS Converter/1
  Sensor/2(plate_pos) -> plate_pos/1
  Sensor/1(plate_rotM) -> plate_rotM/1
  Sensor/3(plate_tilt) -> plate_tilt/1
  Sensor/7(ball_plate_pos) -> ball_plate_pos/1
  Sensor/8(obstacle_distance) -> obstacle_dist/1
  Sensor/9(direction_to_obstacle) -> direction_to_obstacle/1
  Sensor/10(obstacle_x) -> obstacle_x/1
  Sensor/11(obstacle_y) -> obstacle_y/1
  connections:
  Base/LConn1 -- CAD World Frame/RConn1 -- Solver Configuration/RConn1 -- CAD_WF-To-MOAB_WF/LConn1 -- MechanismConfiguration/RConn1
  Sensor/LConn2 -- 6-DOF Joint Plate/RConn1 -- Plate/RConn3
  Spatial Contact Force/LConn1 -- Plate/RConn2
  Plate/LConn1 -- Arm 1/RConn1
  Arm 2/RConn1 -- Plate/LConn2
  Arm 3/RConn1 -- Plate/LConn3
  Sensor/LConn1 -- Ball/RConn1
  Spatial Contact Force/RConn1 -- Ball/LConn1
  Motor 1/LConn1 -- Arm 1/LConn1
  Simulink-PS Converter/RConn1 -- Motor 1/LConn2
  Motor 1/RConn1 -- Base/RConn1
  Arm 2/LConn1 -- Motor 2/LConn1
  Simulink-PS Converter1/RConn1 -- Motor 2/LConn2
  Motor 2/RConn1 -- Base/RConn2
  Arm 3/LConn1 -- Motor 3/LConn1
  Motor 3/LConn2 -- Simulink-PS Converter2/RConn1
  Motor 3/RConn1 -- Base/RConn3
  6-DOF Joint Plate/LConn1 -- CAD_WF-To-MOAB_WF/RConn1

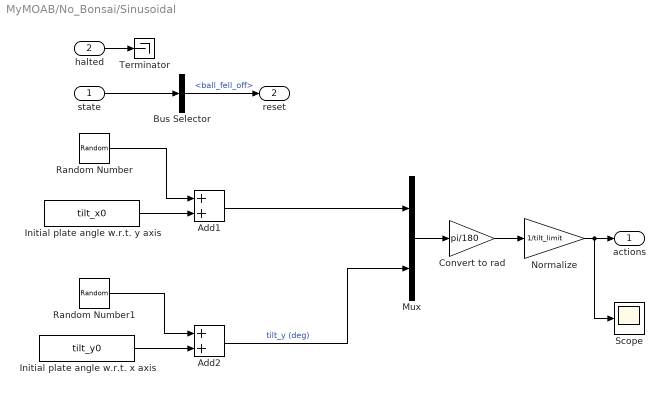
== system MyMOAB/No_Bonsai/Sinusoidal  ==
  state : Inport
  halted : Inport  Port=2
  Add1 : Sum
  Add2 : Sum
  Bus Selector : BusSelector  OutputSignals=ball_fell_off
  Convert to rad : Gain  Gain=pi/180
  Initial plate angle w.r.t. x axis : Constant  Value=tilt_y0
  Initial plate angle w.r.t. y axis : Constant  Value=tilt_x0
  Mux : Mux  Inputs=2
  Normalize : Gain  Gain=1/tilt_limit
  Random Number : RandomNumber  Variance=0.5  SampleTime=DEFAULT_SIMULATION_RATE
  Random Number1 : RandomNumber  Variance=0.5  SampleTime=DEFAULT_SIMULATION_RATE
  Scope : Scope
  Terminator : Terminator
  actions : Outport
  reset : Outport  Port=2
  wires:
  Bus Selector/1 -> reset/1  "<ball_fell_off>"
  Initial plate angle w.r.t. y axis/1 -> Add1/2
  Initial plate angle w.r.t. x axis/1 -> Add2/2
  state/1 -> Bus Selector/1
  halted/1 -> Terminator/1
  Mux/1 -> Convert to rad/1
  Convert to rad/1 -> Normalize/1
  Normalize/1 -> Scope/1, actions/1
  Random Number/1 -> Add1/1
  Random Number1/1 -> Add2/1
  Add2/1 -> Mux/2  "tilt_y (deg)"
  Add1/1 -> Mux/1

== system MyMOAB/MOAB/Iteration Data/Iteration Counter ==
  Constant : Constant  SampleTime=DEFAULT_SIMULATION_RATE
  Counter : Subsystem
  iter : Outport
  wires:
  Constant/1 -> Counter/Enable
  Counter/1(iter) -> iter/1

== system MyMOAB/MOAB/Iteration Data/Subsystem ==
  mode : Inport
  dist_in : Inport  Port=2
  dirn_in : Inport  Port=3
  ox_in : Inport  Port=4
  oy_in : Inport  Port=5
  Product{,1..3} (4 alike) : Product
  dist : Outport
  dirn : Outport  Port=2
  ox : Outport  Port=3
  oy : Outport  Port=4
  wires:
  dist_in/1 -> Product/2
  Product/1 -> dist/1
  Product1/1 -> dirn/1
  dirn_in/1 -> Product1/2
  mode/1 -> Product2/1, Product3/1, Product1/1, Product/1
  ox_in/1 -> Product2/2
  Product2/1 -> ox/1
  oy_in/1 -> Product3/2
  Product3/1 -> oy/1

== system MyMOAB/MOAB/Noise Model/Gaussian Noise ==
  Gain : Gain  Gain=DEFAULT_BALL_NOISE
  Gain1 : Gain  Gain=DEFAULT_PLATE_NOISE
  Gain2 : Gain  Gain=DEFAULT_VEL_NOISE
  Random Number1 : RandomNumber  Mean=noise_mean  Variance=noise_variance
  Random Number2 : RandomNumber  Mean=noise_mean  Variance=noise_variance
  Random Number3 : RandomNumber  Mean=noise_mean  Variance=noise_variance
  plate_noise : Outport
  ball_noise : Outport  Port=2
  vel_noise : Outport  Port=3
  wires:
  Gain/1 -> ball_noise/1
  Random Number3/1 -> Gain2/1
  Random Number2/1 -> Gain/1
  Gain2/1 -> vel_noise/1
  Random Number1/1 -> Gain1/1
  Gain1/1 -> plate_noise/1

== system MyMOAB/MOAB/Noise Model/Zero Noise ==
  Constant : Constant  Value=0
  Constant1 : Constant  Value=0
  Constant2 : Constant  Value=0
  Gain : Gain  Gain=DEFAULT_BALL_NOISE
  Gain1 : Gain  Gain=DEFAULT_PLATE_NOISE
  Gain2 : Gain  Gain=DEFAULT_VEL_NOISE
  plate_noise : Outport
  ball_noise : Outport  Port=2
  vel_noise : Outport  Port=3
  wires:
  Constant1/1 -> Gain/1
  Gain/1 -> ball_noise/1
  Gain1/1 -> plate_noise/1
  Constant2/1 -> Gain2/1
  Constant/1 -> Gain1/1
  Gain2/1 -> vel_noise/1

== system MyMOAB/MOAB/Simscape Model/Arm 1 ==
  Lower Arm : Subsystem
      mask Display: image('MOAB_Arm_Lower_IMAGE.png');
  Magnet : Subsystem
      mask Display: image('MOAB_Arm_Magnet_IMAGE.png');
  Pin : Subsystem
      mask Display: image('MOAB_Arm_Pin_IMAGE.png');
  Revolute Arm : sm_lib/Joints/Revolute Joint  JointMode=Normal  SenseConstraintForce=off  SenseConstraintForceX=off  SenseConstraintForceY=off  SenseConstraintForceZ=off  SenseConstraintTorque=off  SenseConstraintTorqueX=off  SenseConstraintTorqueY=off  SenseConstraintTorqueZ=off  SenseTotalForce=off  SenseTotalForceX=off  SenseTotalForceY=off  SenseTotalForceZ=off  SenseTotalTorque=off  SenseTotalTorqueX=off  SenseTotalTorqueY=off  SenseTotalTorqueZ=off  CompositeWrenchDir=FollowerOnBase  CompositeWrenchFrame=BaseFrame  EquilibriumPosition=0  EquilibriumPositionUnits=rad  SpringStiffness=0  SpringStiffnessUnits=N*m/rad  DampingCoefficient=0  DampingCoefficientUnits=N*m/(rad/s)  TorqueActuationMode=NoTorque  MotionActuationMode=ComputedMotion  SensePosition=off  SenseVelocity=off  SenseAcceleration=off  SenseTorqueForce=off  SenseLowerLimitTorqueForce=off  SenseUpperLimitTorqueForce=off  LowerLimitSpecify=off  LowerLimitBound=-165  LowerLimitBoundUnits=deg  LowerLimitStiffness=1  LowerLimitStiffnessUnits=N*m/deg  LowerLimitDamping=0  LowerLimitDampingUnits=N*m/(deg/s)  LowerLimitTransitionRegionWidth=0.1  LowerLimitTransitionRegionWidthUnits=deg  UpperLimitSpecify=off  UpperLimitBound=0  UpperLimitBoundUnits=deg  UpperLimitStiffness=1  UpperLimitStiffnessUnits=N*m/deg  UpperLimitDamping=0  UpperLimitDampingUnits=N*m/(deg/s)  UpperLimitTransitionRegionWidth=0.1  UpperLimitTransitionRegionWidthUnits=deg  PositionTargetSpecify=off  PositionTargetPriority=Low  PositionTargetValue=45  PositionTargetValueUnits=deg  VelocityTargetSpecify=off  VelocityTargetPriority=High  VelocityTargetValue=0  VelocityTargetValueUnits=deg/s
  Spherical Pin Magnet : sm_lib/Joints/Spherical Joint  JointMode=Normal  SenseConstraintForce=off  SenseConstraintForceX=off  SenseConstraintForceY=off  SenseConstraintForceZ=off  SenseConstraintTorque=off  SenseConstraintTorqueX=off  SenseConstraintTorqueY=off  SenseConstraintTorqueZ=off  SenseTotalForce=off  SenseTotalForceX=off  SenseTotalForceY=off  SenseTotalForceZ=off  SenseTotalTorque=off  SenseTotalTorqueX=off  SenseTotalTorqueY=off  SenseTotalTorqueZ=off  CompositeWrenchDir=FollowerOnBase  CompositeWrenchFrame=BaseFrame  DefPosRotationMethod=None  DefPosRotationAngleUnits=deg  DefPosRotationStandardAxis=+Z  DefPosRotationAngle=0.0  DefPosRotationArbitraryAxis=[0 0 1]  DefPosFollAlignAxisA=+X  DefPosBaseAlignAxisA=+Y  DefPosFollAlignAxisB=+Y  DefPosBaseAlignAxisB=+Z  DefPosRotationSequenceAxes=FollowerAxes  DefPosRotationSequence=XYX  DefPosRotationSequenceAngles=[0 0 0]  DefPosRotationSequenceAnglesUnits=deg  DefPosRotationMatrix=[1 0 0; 0 1 0; 0 0 1]  EqPosRotationMethod=None  EqPosRotationAngleUnits=deg  EqPosRotationStandardAxis=+Z  EqPosRotationAngle=0.0  EqPosRotationArbitraryAxis=[0 0 1]  EqPosFollAlignAxisA=+X  EqPosBaseAlignAxisA=+Y  EqPosFollAlignAxisB=+Y  EqPosBaseAlignAxisB=+Z  EqPosRotationSequenceAxes=FollowerAxes  EqPosRotationSequence=XYX  EqPosRotationSequenceAngles=[0 0 0]  EqPosRotationSequenceAnglesUnits=deg  EqPosRotationMatrix=[1 0 0; 0 1 0; 0 0 1]  SpringStiffness=0  SpringStiffnessUnits=N*m/rad  DampingCoefficient=0  DampingCoefficientUnits=N*m/(rad/s)  ActuateTorqueX=off  ActuateTorqueY=off  ActuateTorqueZ=off  ActuateTorque=off  TorqueActuationMode=NoTorque  MotionActuationMode=ComputedMotion  ActuationFrame=BaseFrame  SensePosition=off  SenseVelocityX=off  SenseVelocityY=off  SenseVelocityZ=off  SenseVelocity=off  SenseAccelerationX=off  SenseAccelerationY=off  SenseAccelerationZ=off  SenseAcceleration=off  SenseTorqueX=off  SenseTorqueY=off  SenseTorqueZ=off  SenseTorqueForce=off  SenseLowerLimitTorqueMag=off  SenseUpperLimitTorqueMag=off  SensingFrame=FollowerFrame  LowerLimitSpecify=off  LowerLimitBound=15  LowerLimitBoundUnits=deg  LowerLimitStiffness=1e4  LowerLimitStiffnessUnits=N*m/deg  LowerLimitDamping=10  LowerLimitDampingUnits=N*m/(deg/s)  LowerLimitTransitionRegionWidth=0.1  LowerLimitTransitionRegionWidthUnits=deg  UpperLimitSpecify=off  UpperLimitBound=45  UpperLimitBoundUnits=deg  UpperLimitStiffness=1e4  UpperLimitStiffnessUnits=N*m/deg  UpperLimitDamping=10  UpperLimitDampingUnits=N*m/(deg/s)  UpperLimitTransitionRegionWidth=0.1  UpperLimitTransitionRegionWidthUnits=deg  PositionTargetRotationMethod=None  PositionTargetRotationAngleUnits=deg  PositionTargetRotationStandardAxis=+Z  PositionTargetRotationAngle=0.0  PositionTargetRotationArbitraryAxis=[0 0 1]  PositionTargetFollAlignAxisA=+X  PositionTargetBaseAlignAxisA=+Y  PositionTargetFollAlignAxisB=+Y  PositionTargetBaseAlignAxisB=+Z  PositionTargetRotationSequenceAxes=FollowerAxes  PositionTargetRotationSequence=XYX  PositionTargetRotationSequenceAngles=[0 0 0]  PositionTargetRotationSequenceAnglesUnits=deg  PositionTargetRotationMatrix=[1 0 0; 0 1 0; 0 0 1]  PositionTargetSpecify=off  PositionTargetPriority=High  VelocityTargetValue=[0 0 0]  VelocityTargetValueUnits=deg/s  VelocityTargetSpecify=off  VelocityTargetPriority=High  VelocityTargetInFollowerFrame=on
  Upper Arm : Subsystem
      mask Display: image('MOAB_Arm_Upper_IMAGE.png');
  F : PMIOPort  Side=Right
  B : PMIOPort  Port=2  Side=Left
  connections:
  B/RConn1 -- Lower Arm/RConn1
  Lower Arm/LConn1 -- Revolute Arm/RConn1
  Magnet/RConn1 -- Spherical Pin Magnet/LConn1
  Pin/RConn1 -- Spherical Pin Magnet/RConn1
  F/RConn1 -- Magnet/LConn1
  Upper Arm/LConn1 -- Revolute Arm/LConn1
  Upper Arm/RConn1 -- Pin/LConn1

== system MyMOAB/MOAB/Simscape Model/Arm 2 ==
  Lower Arm : Subsystem
      mask Display: image('MOAB_Arm_Lower_IMAGE.png');
  Magnet : Subsystem
      mask Display: image('MOAB_Arm_Magnet_IMAGE.png');
  Pin : Subsystem
      mask Display: image('MOAB_Arm_Pin_IMAGE.png');
  Revolute Arm : sm_lib/Joints/Revolute Joint  JointMode=Normal  SenseConstraintForce=off  SenseConstraintForceX=off  SenseConstraintForceY=off  SenseConstraintForceZ=off  SenseConstraintTorque=off  SenseConstraintTorqueX=off  SenseConstraintTorqueY=off  SenseConstraintTorqueZ=off  SenseTotalForce=off  SenseTotalForceX=off  SenseTotalForceY=off  SenseTotalForceZ=off  SenseTotalTorque=off  SenseTotalTorqueX=off  SenseTotalTorqueY=off  SenseTotalTorqueZ=off  CompositeWrenchDir=FollowerOnBase  CompositeWrenchFrame=BaseFrame  EquilibriumPosition=0  EquilibriumPositionUnits=rad  SpringStiffness=0  SpringStiffnessUnits=N*m/rad  DampingCoefficient=0  DampingCoefficientUnits=N*m/(rad/s)  TorqueActuationMode=NoTorque  MotionActuationMode=ComputedMotion  SensePosition=off  SenseVelocity=off  SenseAcceleration=off  SenseTorqueForce=off  SenseLowerLimitTorqueForce=off  SenseUpperLimitTorqueForce=off  LowerLimitSpecify=off  LowerLimitBound=-165  LowerLimitBoundUnits=deg  LowerLimitStiffness=1  LowerLimitStiffnessUnits=N*m/deg  LowerLimitDamping=0  LowerLimitDampingUnits=N*m/(deg/s)  LowerLimitTransitionRegionWidth=0.1  LowerLimitTransitionRegionWidthUnits=deg  UpperLimitSpecify=off  UpperLimitBound=0  UpperLimitBoundUnits=deg  UpperLimitStiffness=1  UpperLimitStiffnessUnits=N*m/deg  UpperLimitDamping=0  UpperLimitDampingUnits=N*m/(deg/s)  UpperLimitTransitionRegionWidth=0.1  UpperLimitTransitionRegionWidthUnits=deg  PositionTargetSpecify=off  PositionTargetPriority=Low  PositionTargetValue=45  PositionTargetValueUnits=deg  VelocityTargetSpecify=off  VelocityTargetPriority=High  VelocityTargetValue=0  VelocityTargetValueUnits=deg/s
  Spherical Pin Magnet : sm_lib/Joints/Spherical Joint  JointMode=Normal  SenseConstraintForce=off  SenseConstraintForceX=off  SenseConstraintForceY=off  SenseConstraintForceZ=off  SenseConstraintTorque=off  SenseConstraintTorqueX=off  SenseConstraintTorqueY=off  SenseConstraintTorqueZ=off  SenseTotalForce=off  SenseTotalForceX=off  SenseTotalForceY=off  SenseTotalForceZ=off  SenseTotalTorque=off  SenseTotalTorqueX=off  SenseTotalTorqueY=off  SenseTotalTorqueZ=off  CompositeWrenchDir=FollowerOnBase  CompositeWrenchFrame=BaseFrame  DefPosRotationMethod=None  DefPosRotationAngleUnits=deg  DefPosRotationStandardAxis=+Z  DefPosRotationAngle=0.0  DefPosRotationArbitraryAxis=[0 0 1]  DefPosFollAlignAxisA=+X  DefPosBaseAlignAxisA=+Y  DefPosFollAlignAxisB=+Y  DefPosBaseAlignAxisB=+Z  DefPosRotationSequenceAxes=FollowerAxes  DefPosRotationSequence=XYX  DefPosRotationSequenceAngles=[0 0 0]  DefPosRotationSequenceAnglesUnits=deg  DefPosRotationMatrix=[1 0 0; 0 1 0; 0 0 1]  EqPosRotationMethod=None  EqPosRotationAngleUnits=deg  EqPosRotationStandardAxis=+Z  EqPosRotationAngle=0.0  EqPosRotationArbitraryAxis=[0 0 1]  EqPosFollAlignAxisA=+X  EqPosBaseAlignAxisA=+Y  EqPosFollAlignAxisB=+Y  EqPosBaseAlignAxisB=+Z  EqPosRotationSequenceAxes=FollowerAxes  EqPosRotationSequence=XYX  EqPosRotationSequenceAngles=[0 0 0]  EqPosRotationSequenceAnglesUnits=deg  EqPosRotationMatrix=[1 0 0; 0 1 0; 0 0 1]  SpringStiffness=0  SpringStiffnessUnits=N*m/rad  DampingCoefficient=0  DampingCoefficientUnits=N*m/(rad/s)  ActuateTorqueX=off  ActuateTorqueY=off  ActuateTorqueZ=off  ActuateTorque=off  TorqueActuationMode=NoTorque  MotionActuationMode=ComputedMotion  ActuationFrame=BaseFrame  SensePosition=off  SenseVelocityX=off  SenseVelocityY=off  SenseVelocityZ=off  SenseVelocity=off  SenseAccelerationX=off  SenseAccelerationY=off  SenseAccelerationZ=off  SenseAcceleration=off  SenseTorqueX=off  SenseTorqueY=off  SenseTorqueZ=off  SenseTorqueForce=off  SenseLowerLimitTorqueMag=off  SenseUpperLimitTorqueMag=off  SensingFrame=FollowerFrame  LowerLimitSpecify=off  LowerLimitBound=15  LowerLimitBoundUnits=deg  LowerLimitStiffness=1e4  LowerLimitStiffnessUnits=N*m/deg  LowerLimitDamping=10  LowerLimitDampingUnits=N*m/(deg/s)  LowerLimitTransitionRegionWidth=0.1  LowerLimitTransitionRegionWidthUnits=deg  UpperLimitSpecify=off  UpperLimitBound=45  UpperLimitBoundUnits=deg  UpperLimitStiffness=1e4  UpperLimitStiffnessUnits=N*m/deg  UpperLimitDamping=10  UpperLimitDampingUnits=N*m/(deg/s)  UpperLimitTransitionRegionWidth=0.1  UpperLimitTransitionRegionWidthUnits=deg  PositionTargetRotationMethod=None  PositionTargetRotationAngleUnits=deg  PositionTargetRotationStandardAxis=+Z  PositionTargetRotationAngle=0.0  PositionTargetRotationArbitraryAxis=[0 0 1]  PositionTargetFollAlignAxisA=+X  PositionTargetBaseAlignAxisA=+Y  PositionTargetFollAlignAxisB=+Y  PositionTargetBaseAlignAxisB=+Z  PositionTargetRotationSequenceAxes=FollowerAxes  PositionTargetRotationSequence=XYX  PositionTargetRotationSequenceAngles=[0 0 0]  PositionTargetRotationSequenceAnglesUnits=deg  PositionTargetRotationMatrix=[1 0 0; 0 1 0; 0 0 1]  PositionTargetSpecify=off  PositionTargetPriority=High  VelocityTargetValue=[0 0 0]  VelocityTargetValueUnits=deg/s  VelocityTargetSpecify=off  VelocityTargetPriority=High  VelocityTargetInFollowerFrame=on
  Upper Arm : Subsystem
      mask Display: image('MOAB_Arm_Upper_IMAGE.png');
  F : PMIOPort  Side=Right
  B : PMIOPort  Port=2  Side=Left
  connections:
  Magnet/RConn1 -- Spherical Pin Magnet/LConn1
  F/RConn1 -- Magnet/LConn1
  Upper Arm/RConn1 -- Pin/LConn1
  Upper Arm/LConn1 -- Revolute Arm/LConn1
  Lower Arm/LConn1 -- Revolute Arm/RConn1
  Pin/RConn1 -- Spherical Pin Magnet/RConn1
  B/RConn1 -- Lower Arm/RConn1
